simulink model "Integration4"  (R2025a)
settings: Solver=ode113  StartTime=0.0  StopTime=7200  FixedStep=1e-04  MaxStep=72  RelTol=1e-3
libraries: simulink x3302
(part 1 of 141)
settings Model: Creator=kbiswas  LastModifiedBy=kaust
settings RTWCC: GPUComputeCapability=3.5

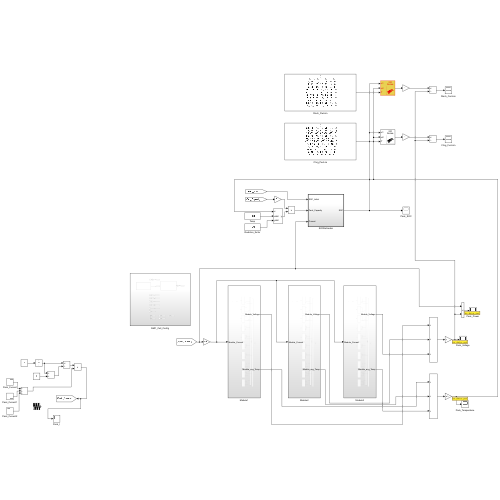
[thumbnail: Simulink's stored preview of the top-level diagram]
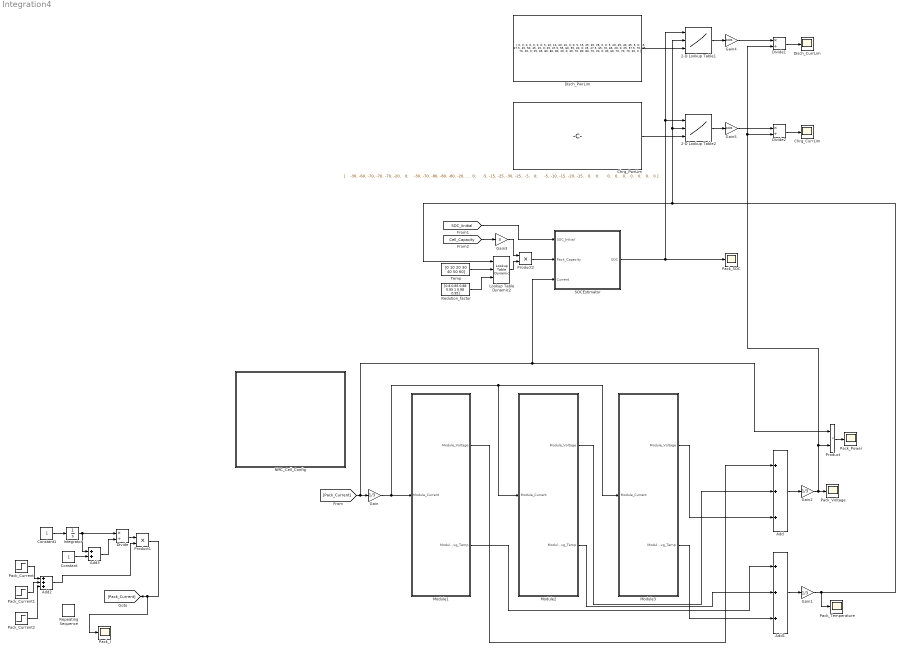
== system Integration4 ==
  2-D Lookup Table1 : Lookup_n-D  LookupTableObject=''  BreakpointsForDimension1=[0 0.1 0.2 0.3 0.4 0.5 0.6 0.7 0.8 0.9 1]  BreakpointsForDimension2=[0 10 20 30 40 50 60]  BreakpointsForDimension1FirstPoint=10  BreakpointsForDimension2FirstPoint=10  BreakpointsForDimension1Spacing=12  BreakpointsForDimension2Spacing=12  IndexSearchMethod=Evenly spaced points  TableSource=Input port  Table=|  InterpMethod=Akima spline  DiagnosticForOutOfRangeInput=Error  InternalRulePriority=Speed  RndMeth=Simplest
      | [
      |     2.954364, 3.109857, 3.273534, 3.3066, 3.34,    3.3734,  3.20473;
      |     3.122427, 3.286765, 3.459753, 3.4947, 3.53,    3.5653,  3.387035;
      |     3.175499, 3.342631, 3.518559, 3.5541, 3.59,    3.6259,  3.444605;
      |     3.210881, 3.379875, 3.557763, 3.5937, 3.63,    3.6663,  3.482985;
      |     3.237417, 3.407808, 3.587166, 3.6234, 3.66,    3.6966,  3.511777;
      |     3.272799, 3.445052, 3.62637,  3.663,  3.7,     3.737,   3.55015;
      |     3.317026, 3.491066, 3.675375, 3.7125, 3.75,    3.7875,  3.598125;
      |     3.387789, 3.566094, 3.753783, 3.7917, 3.83,    3.8683,  3.674885;
      |     3.467398, 3.649892, 3.841992, 3.8808, 3.92,    3.9592,  3.76124;
      |     3.564697, 3.752313, 3.949803, 3.9897, 4.03,    4.0703,  3.866785;
      |     3.653151, 3.845422, 4.047813, 4.0887, 4.13,    4.1713,  3.962735
      | ]
      settings: InputPortMap=u0,u1,p221
  2-D Lookup Table2 : Lookup_n-D  LookupTableObject=''  BreakpointsForDimension1=[0 0.1 0.2 0.3 0.4 0.5 0.6 0.7 0.8 0.9 1]  BreakpointsForDimension2=[0 10 20 30 40 50 60]  BreakpointsForDimension1FirstPoint=10  BreakpointsForDimension2FirstPoint=10  BreakpointsForDimension1Spacing=12  BreakpointsForDimension2Spacing=12  IndexSearchMethod=Evenly spaced points  TableSource=Input port  Table=|  InterpMethod=Akima spline  DiagnosticForOutOfRangeInput=Error  InternalRulePriority=Speed  RndMeth=Simplest
      | [
      |     2.954364, 3.109857, 3.273534, 3.3066, 3.34,    3.3734,  3.20473;
      |     3.122427, 3.286765, 3.459753, 3.4947, 3.53,    3.5653,  3.387035;
      |     3.175499, 3.342631, 3.518559, 3.5541, 3.59,    3.6259,  3.444605;
      |     3.210881, 3.379875, 3.557763, 3.5937, 3.63,    3.6663,  3.482985;
      |     3.237417, 3.407808, 3.587166, 3.6234, 3.66,    3.6966,  3.511777;
      |     3.272799, 3.445052, 3.62637,  3.663,  3.7,     3.737,   3.55015;
      |     3.317026, 3.491066, 3.675375, 3.7125, 3.75,    3.7875,  3.598125;
      |     3.387789, 3.566094, 3.753783, 3.7917, 3.83,    3.8683,  3.674885;
      |     3.467398, 3.649892, 3.841992, 3.8808, 3.92,    3.9592,  3.76124;
      |     3.564697, 3.752313, 3.949803, 3.9897, 4.03,    4.0703,  3.866785;
      |     3.653151, 3.845422, 4.047813, 4.0887, 4.13,    4.1713,  3.962735
      | ]
      settings: InputPortMap=u0,u1,p221
  Add : Sum  Inputs=+++
  Add1 : Sum  Inputs=+++
  Add2 : Sum  Inputs=+++
  Add3 : Sum
  Chrg_CurrLim : Scope
      settings: ActiveDisplayYMinimum=-0.029859398179627156  ActiveDisplayYMaximum=1.1144288220199585  DataLoggingVariableName=ScopeData8
  Chrg_PwrLim : Constant  Value=|
      | [
      |    -30, -60, -70, -70, -70, -20,   0;
      |    -30, -70, -80, -80, -80, -20,   0;
      |    -25, -65, -80, -80, -80, -20,   0;
      |    -25, -55, -70, -75, -70, -20,   0;
      |    -25, -47.5, -65, -70, -65, -20,  0;
      |    -25, -37.5, -55, -60, -55, -20,  0;
      |    -15, -27.5, -45, -50, -45, -15,  0;
      |     -5, -20, -35, -40, -35,  -5,   0;
      |     -5, -15, -25, -30, -25,  -5,   0;
      |     -5, -10, -15, -20, -15,   0,   0;
      |      0,   0,   0,   0,   0,   0,   0
      | ]
  Constant : Constant
  Constant1 : Constant
  Disch_CurrLim : Scope
      settings: ActiveDisplayYMinimum=-0.029859398179627156  ActiveDisplayYMaximum=1.1144288220199585  DataLoggingVariableName=ScopeData7
  Disch_PwrLim : Constant  Value=|
      | [
      |      0,   0,   0,   0,   0,   0,   0;
      |      5,  10,  10,  20,  10,   0,   0;
      |      5,  15,  25,  30,  25,   5,   0;
      |      5,  20,  35,  40,  35,   5,   0;
      |     15, 27.5, 45,  50,  45,  15,   0;
      |     25, 37.5, 55,  60,  55,  20,   0;
      |     25, 47.5, 65,  70,  65,  20,   0;
      |     25, 57.5, 70,  75,  70,  20,   0;
      |     25, 65,   80,  80,  80,  20,   0;
      |     30, 70,   80,  80,  70,  20,   0;
      |     30, 60,   70,  70,  70,  20,   0
      | ]
  Divide : Product  Inputs=*/
  Divide1 : Product  Inputs=*/
  Divide2 : Product  Inputs=*/
  Gain : Gain  Gain=1/3
  Gain1 : Gain  Gain=1/3
  Gain2 : Gain  Gain=1/3
  Gain3 : Gain  Gain=3
  Gain4 : Gain  Gain=1000
  Gain5 : Gain  Gain=1000
  Integrator : Integrator
  Lookup Table Dynamic2 : simulink/Lookup Tables/Lookup Table Dynamic  LookUpMeth=Interpolation-Use End Values  OutDataType=fixdt('double')  OutScaling=[]  OutputDataTypeScalingMode=Specify via dialog  OutDataTypeStr=fixdt('double')  DoSatur=off
  Module1 : Subsystem
  Module2 : Subsystem
  Module3 : Subsystem
  NMC_Cell_Config : Subsystem
  Pack_Current : Step  After=70  SampleTime=0
  Pack_Current1 : Step  Time=3601  After=-70  SampleTime=0
  Pack_Current2 : Step  Time=3610  After=-70  SampleTime=0
  Pack_I : Scope
      settings: ActiveDisplayYMinimum=-87.4866348128896  ActiveDisplayYMaximum=87.47692203701736  DataLoggingVariableName=ScopeData5
  Pack_Power : Scope
      settings: ActiveDisplayYMinimum=-86878.920066941544  ActiveDisplayYMaximum=76635.6657175614  DataLoggingVariableName=ScopeData4
  Pack_SOC : Scope
      settings: ActiveDisplayYMinimum=-0.029859398179627156  ActiveDisplayYMaximum=1.1144288220199585  DataLoggingVariableName=ScopeData6
  Pack_Temperature : Scope
      settings: ActiveDisplayYMinimum=24.036198918147498  ActiveDisplayYMaximum=33.674209736672459  DataLoggingVariableName=ScopeData2
  Pack_Voltage : Scope
      settings: ActiveDisplayYMinimum=715.78941909752871  ActiveDisplayYMaximum=961.19940125009657
  Product : Product
  Product1 : Product
  Product2 : Product
  Redution_factor : Constant  Value=[0.8 0.85 0.88 0.95 1 0.98 0.95]
  Repeating Sequence : simulink/Sources/Repeating Sequence  rep_seq_t=[0 200 400 600 800]  rep_seq_y=[0 70 0 -70 0]
  SOCEstimator : Subsystem  TreatAsAtomicUnit=on
  Temp : Constant  Value=[0 10 20 30 40 50 60]
  wires:
  [Pack_Current] -> Product/1, SOCEstimator/3(Current), Gain/1
  Gain/1 -> Module2/1(Module_Current), Module3/1(Module_Current), Module1/1(Module_Current)
  Module1/1(Module_Voltage) -> Add/1
  Module2/1(Module_Voltage) -> Add/2
  Module3/1(Module_Voltage) -> Add/3
  Module1/2(Module_avg_Temp) -> Add1/1
  Module2/2(Module_avg_Temp) -> Add1/2
  Module3/2(Module_avg_Temp) -> Add1/3
  Add1/1 -> Gain1/1
  Add/1 -> Gain2/1
  Gain2/1 -> Divide2/2, Divide1/2, Product/2, Pack_Voltage/1
  Pack_Current/1 -> Add2/1
  Pack_Current1/1 -> Add2/2
  Product/1 -> Pack_Power/1
  Product1/1 -> Pack_I/1, [Pack_Current]
  Add2/1 -> Product1/2
  Integrator/1 -> Divide/1, Add3/1
  Constant/1 -> Add3/2
  Add3/1 -> Divide/2
  Constant1/1 -> Integrator/1
  Divide/1 -> Product1/1
  Pack_Current2/1 -> Add2/3
  [SOC_Iinitial] -> SOCEstimator/1(SOC_Initial)
  Lookup Table Dynamic2/1 -> Product2/2
  [Cell_Capacity] -> Gain3/1
  Temp/1 -> Lookup Table Dynamic2/2
  Gain1/1 -> 2-D Lookup Table1/2, 2-D Lookup Table2/2, Lookup Table Dynamic2/1, Pack_Temperature/1
  Redution_factor/1 -> Lookup Table Dynamic2/3
  Product2/1 -> SOCEstimator/2(Pack_Capacity)
  Gain3/1 -> Product2/1
  SOCEstimator/1(SOC) -> 2-D Lookup Table2/1, 2-D Lookup Table1/1, Pack_SOC/1
  Disch_PwrLim/1 -> 2-D Lookup Table1/3
  Chrg_PwrLim/1 -> 2-D Lookup Table2/3
  2-D Lookup Table1/1 -> Gain4/1
  2-D Lookup Table2/1 -> Gain5/1
  Gain4/1 -> Divide1/1
  Gain5/1 -> Divide2/1
  Divide1/1 -> Disch_CurrLim/1
  Divide2/1 -> Chrg_CurrLim/1

== system Integration4/Module1 ==
  Module_Current : Inport
  Add : Sum  Inputs=++++++++++
  Add1 : Sum  Inputs=++++++++++
  Constant : Constant  Value=10
  Divide : Product  Inputs=*/
  Scope : Scope
      settings: ActiveDisplayYMinimum=675.19968  ActiveDisplayYMaximum=920.25224
  Scope1 : Scope
      settings: ActiveDisplayYMinimum=23.92172  ActiveDisplayYMaximum=34.70451  DataLoggingVariableName=ScopeData3
  SubModule_1 : Subsystem
  SubModule_10 : Subsystem
  SubModule_2 : Subsystem
  SubModule_3 : Subsystem
  SubModule_4 : Subsystem
  SubModule_5 : Subsystem
  SubModule_6 : Subsystem
  SubModule_7 : Subsystem
  SubModule_8 : Subsystem
  SubModule_9 : Subsystem
  Module_Voltage : Outport
  Module_avg_Temp : Outport  Port=2
  wires:
  SubModule_4/2(SubModule_avg_temp) -> Add1/4
  Add/1 -> Module_Voltage/1, Scope/1
  [Module_Current] -> SubModule_5/1(Module_Current)
  [Module_Current] -> SubModule_9/1(Module_Current)
  [Module_Current] -> SubModule_2/1(Module_Current)
  [Module_Current] -> SubModule_3/1(Module_Current)
  [Module_Current] -> SubModule_7/1(Module_Current)
  Module_Current/1 -> [Module_Current]
  SubModule_1/1(SubModule_Voltage) -> Add/1
  [Module_Current] -> SubModule_1/1(Module_Current)
  [Module_Current] -> SubModule_4/1(Module_Current)
  SubModule_6/2(SubModule_avg_temp) -> Add1/6
  Divide/1 -> Module_avg_Temp/1, Scope1/1
  SubModule_5/1(SubModule_Voltage) -> Add/5
  [Module_Current] -> SubModule_8/1(Module_Current)
  SubModule_8/2(SubModule_avg_temp) -> Add1/8
  SubModule_5/2(SubModule_avg_temp) -> Add1/5
  SubModule_8/1(SubModule_Voltage) -> Add/8
  [Module_Current] -> SubModule_10/1(Module_Current)
  Constant/1 -> Divide/2
  SubModule_10/1(SubModule_Voltage) -> Add/10
  SubModule_10/2(SubModule_avg_temp) -> Add1/10
  SubModule_7/1(SubModule_Voltage) -> Add/7
  SubModule_9/2(SubModule_avg_temp) -> Add1/9
  SubModule_3/1(SubModule_Voltage) -> Add/3
  SubModule_4/1(SubModule_Voltage) -> Add/4
  SubModule_2/2(SubModule_avg_temp) -> Add1/2
  SubModule_3/2(SubModule_avg_temp) -> Add1/3
  SubModule_7/2(SubModule_avg_temp) -> Add1/7
  Add1/1 -> Divide/1
  SubModule_9/1(SubModule_Voltage) -> Add/9
  SubModule_6/1(SubModule_Voltage) -> Add/6
  SubModule_2/1(SubModule_Voltage) -> Add/2
  SubModule_1/2(SubModule_avg_temp) -> Add1/1
  [Module_Current] -> SubModule_6/1(Module_Current)

== system Integration4/Module2 ==
  Module_Current : Inport
  Add : Sum  Inputs=++++++++++
  Add1 : Sum  Inputs=++++++++++
  Constant : Constant  Value=10
  Divide : Product  Inputs=*/
  Scope : Scope
      settings: ActiveDisplayYMinimum=675.19968  ActiveDisplayYMaximum=920.25224
  Scope1 : Scope
      settings: ActiveDisplayYMinimum=23.92172  ActiveDisplayYMaximum=34.70451  DataLoggingVariableName=ScopeData3
  SubModule_1 : Subsystem
  SubModule_10 : Subsystem
  SubModule_2 : Subsystem
  SubModule_3 : Subsystem
  SubModule_4 : Subsystem
  SubModule_5 : Subsystem
  SubModule_6 : Subsystem
  SubModule_7 : Subsystem
  SubModule_8 : Subsystem
  SubModule_9 : Subsystem
  Module_Voltage : Outport
  Module_avg_Temp : Outport  Port=2
  wires:
  SubModule_4/2(SubModule_avg_temp) -> Add1/4
  Add/1 -> Module_Voltage/1, Scope/1
  [Module_Current] -> SubModule_5/1(Module_Current)
  [Module_Current] -> SubModule_9/1(Module_Current)
  [Module_Current] -> SubModule_2/1(Module_Current)
  [Module_Current] -> SubModule_3/1(Module_Current)
  [Module_Current] -> SubModule_7/1(Module_Current)
  Module_Current/1 -> [Module_Current]
  SubModule_1/1(SubModule_Voltage) -> Add/1
  [Module_Current] -> SubModule_1/1(Module_Current)
  [Module_Current] -> SubModule_4/1(Module_Current)
  SubModule_6/2(SubModule_avg_temp) -> Add1/6
  Divide/1 -> Module_avg_Temp/1, Scope1/1
  SubModule_5/1(SubModule_Voltage) -> Add/5
  [Module_Current] -> SubModule_8/1(Module_Current)
  SubModule_8/2(SubModule_avg_temp) -> Add1/8
  SubModule_5/2(SubModule_avg_temp) -> Add1/5
  SubModule_8/1(SubModule_Voltage) -> Add/8
  [Module_Current] -> SubModule_10/1(Module_Current)
  Constant/1 -> Divide/2
  SubModule_10/1(SubModule_Voltage) -> Add/10
  SubModule_10/2(SubModule_avg_temp) -> Add1/10
  SubModule_7/1(SubModule_Voltage) -> Add/7
  SubModule_9/2(SubModule_avg_temp) -> Add1/9
  SubModule_3/1(SubModule_Voltage) -> Add/3
  SubModule_4/1(SubModule_Voltage) -> Add/4
  SubModule_2/2(SubModule_avg_temp) -> Add1/2
  SubModule_3/2(SubModule_avg_temp) -> Add1/3
  SubModule_7/2(SubModule_avg_temp) -> Add1/7
  Add1/1 -> Divide/1
  SubModule_9/1(SubModule_Voltage) -> Add/9
  SubModule_6/1(SubModule_Voltage) -> Add/6
  SubModule_2/1(SubModule_Voltage) -> Add/2
  SubModule_1/2(SubModule_avg_temp) -> Add1/1
  [Module_Current] -> SubModule_6/1(Module_Current)

== system Integration4/Module3 ==
  Module_Current : Inport
  Add : Sum  Inputs=++++++++++
  Add1 : Sum  Inputs=++++++++++
  Constant : Constant  Value=10
  Divide : Product  Inputs=*/
  Scope : Scope
      settings: ActiveDisplayYMinimum=618.46252  ActiveDisplayYMaximum=926.55637
  Scope1 : Scope
      settings: ActiveDisplayYMinimum=23.92172  ActiveDisplayYMaximum=34.70451  DataLoggingVariableName=ScopeData3
  SubModule_1 : Subsystem
  SubModule_10 : Subsystem
  SubModule_2 : Subsystem
  SubModule_3 : Subsystem
  SubModule_4 : Subsystem
  SubModule_5 : Subsystem
  SubModule_6 : Subsystem
  SubModule_7 : Subsystem
  SubModule_8 : Subsystem
  SubModule_9 : Subsystem
  Module_Voltage : Outport
  Module_avg_Temp : Outport  Port=2
  wires:
  [Module_Current] -> SubModule_6/1(Module_Current)
  SubModule_1/2(SubModule_avg_temp) -> Add1/1
  SubModule_2/1(SubModule_Voltage) -> Add/2
  SubModule_6/1(SubModule_Voltage) -> Add/6
  SubModule_9/1(SubModule_Voltage) -> Add/9
  Add1/1 -> Divide/1
  SubModule_7/2(SubModule_avg_temp) -> Add1/7
  SubModule_3/2(SubModule_avg_temp) -> Add1/3
  SubModule_2/2(SubModule_avg_temp) -> Add1/2
  SubModule_4/1(SubModule_Voltage) -> Add/4
  SubModule_3/1(SubModule_Voltage) -> Add/3
  SubModule_9/2(SubModule_avg_temp) -> Add1/9
  SubModule_7/1(SubModule_Voltage) -> Add/7
  SubModule_10/2(SubModule_avg_temp) -> Add1/10
  SubModule_10/1(SubModule_Voltage) -> Add/10
  Constant/1 -> Divide/2
  [Module_Current] -> SubModule_10/1(Module_Current)
  SubModule_8/1(SubModule_Voltage) -> Add/8
  SubModule_5/2(SubModule_avg_temp) -> Add1/5
  SubModule_8/2(SubModule_avg_temp) -> Add1/8
  [Module_Current] -> SubModule_8/1(Module_Current)
  SubModule_5/1(SubModule_Voltage) -> Add/5
  Divide/1 -> Scope1/1, Module_avg_Temp/1
  SubModule_6/2(SubModule_avg_temp) -> Add1/6
  [Module_Current] -> SubModule_4/1(Module_Current)
  [Module_Current] -> SubModule_1/1(Module_Current)
  SubModule_1/1(SubModule_Voltage) -> Add/1
  Module_Current/1 -> [Module_Current]
  [Module_Current] -> SubModule_7/1(Module_Current)
  [Module_Current] -> SubModule_3/1(Module_Current)
  [Module_Current] -> SubModule_2/1(Module_Current)
  [Module_Current] -> SubModule_9/1(Module_Current)
  [Module_Current] -> SubModule_5/1(Module_Current)
  Add/1 -> Scope/1, Module_Voltage/1
  SubModule_4/2(SubModule_avg_temp) -> Add1/4

== system Integration4/NMC_Cell_Config ==
  A : Constant  Value=0.013
  C1_User1 : Constant  Value=[800 850 900 950 1000 1050 1000 950 900 850 800]
  C2_User : Constant  Value=[15 16 17 18 19 20 19 18 17 16 15]
  Cell_Capacity_Ah_rated : Constant  Value=26.5
  Gain1 : Gain  Gain=1e-03
  Gain2 : Gain
  Gain3 : Gain  Gain=1e-03
  Gain4 : Gain  Gain=1e+03
  Gain5 : Gain  Gain=0.01
  Gain6 : Gain  Gain=1e-04
  Goto11 : Goto  TagVisibility=global
  M*Cp : Constant  Value=369
  OCV_NMC : Constant  Value=|
      | [
      |     2.954364, 3.109857, 3.273534, 3.3066, 3.34,    3.3734,  3.20473;
      |     3.122427, 3.286765, 3.459753, 3.4947, 3.53,    3.5653,  3.387035;
      |     3.175499, 3.342631, 3.518559, 3.5541, 3.59,    3.6259,  3.444605;
      |     3.210881, 3.379875, 3.557763, 3.5937, 3.63,    3.6663,  3.482985;
      |     3.237417, 3.407808, 3.587166, 3.6234, 3.66,    3.6966,  3.511777;
      |     3.272799, 3.445052, 3.62637,  3.663,  3.7,     3.737,   3.55015;
      |     3.317026, 3.491066, 3.675375, 3.7125, 3.75,    3.7875,  3.598125;
      |     3.387789, 3.566094, 3.753783, 3.7917, 3.83,    3.8683,  3.674885;
      |     3.467398, 3.649892, 3.841992, 3.8808, 3.92,    3.9592,  3.76124;
      |     3.564697, 3.752313, 3.949803, 3.9897, 4.03,    4.0703,  3.866785;
      |     3.653151, 3.845422, 4.047813, 4.0887, 4.13,    4.1713,  3.962735
      | ]
  R1_User : Constant  Value=[1.5 1.2 0.9 0.7 0.6 0.5 0.5 0.5 0.6 0.7 0.8]
  R2_User1 : Constant  Value=[2.5 2 1.6 1.3 1.1 1 1.1 1.2 1.3 1.4 1.5]
  Ri_NMC : Constant  Value=|
      | [67.2155, 61.105, 55.55, 55, 52.25, 49.6375, 54.60125;
      |     48.884, 44.44, 40.4, 40, 38, 36.1, 39.71;
      |     44.60665, 40.5515, 36.865, 36.5, 34.675, 32.94125, 36.23538;
      |     41.5514, 37.774, 34.34, 34, 32.83, 30.685, 33.7535;
      |     40.3293, 36.663, 33.33, 33, 31.35, 29.7825, 32.76075;
      |     39.71825, 36.1075, 32.825, 32.5, 31.25, 29.33125, 32.26438;
      |     40.08488, 36.4408, 33.128, 32.8, 31.16, 29.602, 32.5622;
      |     40.94035, 37.2185, 33.835, 33.5, 31.825, 30.23375, 33.15738;
      |     42.7735, 38.1925, 35.03, 34.7, 32.375, 31.5875, 34.74263;
      |     51.3282, 46.602, 42.42, 42, 39.9, 37.905, 41.6955;
      |     73.326, 66.66, 60.6, 60, 57, 54.15, 59.565]
  SOC_Initial_% : Constant  Value=100
  SOC_User : Constant  Value=[0 10 20 30 40 50 60 70 80 90 100]
  Temp_Initial_degC : Constant  Value=25
  Temp_ambient : Constant  Value=25
  h : Constant  Value=20
  tag scope: C1_User=global, C2_User=global, Cell_Capacity=global, Cp=global, OCV=global, R1_User=global, R2_User=global, Ri_User=global, SOC_Iinitial=global, SOC_User=global, Temp_Iinitial=global, Temp_ambient=global, h=global
  wires:
  OCV_NMC/1 -> [OCV]
  SOC_User/1 -> Gain5/1
  R1_User/1 -> Gain1/1
  Gain1/1 -> [R1_User]
  C1_User1/1 -> Gain2/1
  Gain2/1 -> [C1_User]
  R2_User1/1 -> Gain3/1
  Gain3/1 -> [R2_User]
  Gain4/1 -> [C2_User]
  C2_User/1 -> Gain4/1
  Cell_Capacity_Ah_rated/1 -> [Cell_Capacity]
  SOC_Initial_%/1 -> [SOC_Iinitial]
  Gain5/1 -> [SOC_User]
  Temp_Initial_degC/1 -> [Temp_ambient], [Temp_Iinitial]
  h/1 -> [h]
  A/1 -> Goto11/1
  M*Cp/1 -> [Cp]
  Gain6/1 -> [Ri_User]
  Ri_NMC/1 -> Gain6/1

== system Integration4/SOCEstimator ==
  SOC_Initial : Inport
  Pack_Capacity : Inport  Port=2
  Current : Inport  Port=3
  SOCEstimator : Subsystem
  SOC : Outport
  wires:
  SOCEstimator/1(SOC) -> SOC/1
  SOC_Initial/1 -> SOCEstimator/1(SOC_Initial)
  Current/1 -> SOCEstimator/2(Current)
  Pack_Capacity/1 -> SOCEstimator/3(CellCapacity)

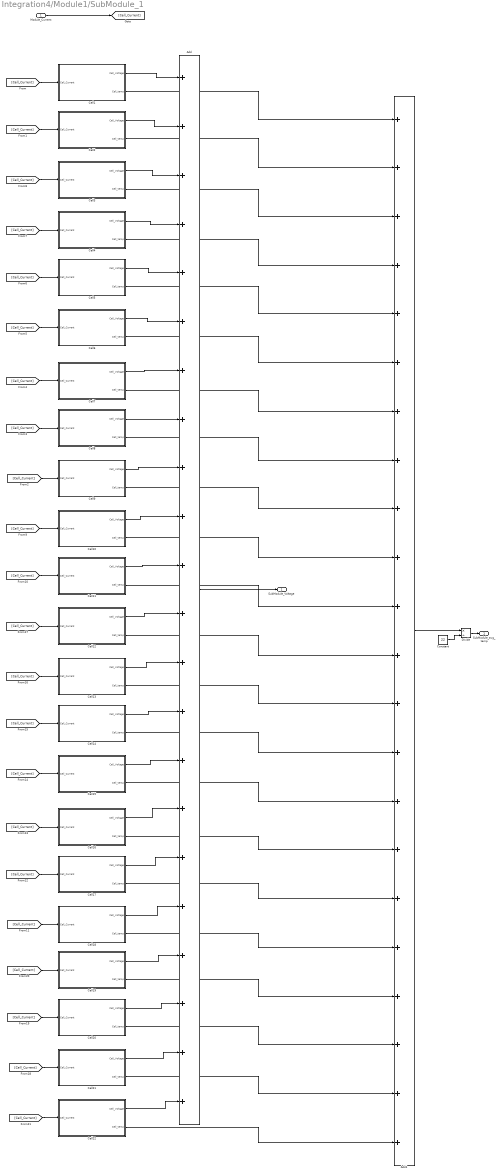
== system Integration4/Module1/SubModule_1 ==
  Module_Current : Inport
  Add : Sum  Inputs=++++++++++++++++++++++
  Add1 : Sum  Inputs=++++++++++++++++++++++
  Cell1 : Subsystem
  Cell10 : Subsystem
  Cell11 : Subsystem
  Cell12 : Subsystem
  Cell13 : Subsystem
  Cell14 : Subsystem
  Cell15 : Subsystem
  Cell16 : Subsystem
  Cell17 : Subsystem
  Cell18 : Subsystem
  Cell19 : Subsystem
  Cell2 : Subsystem
  Cell20 : Subsystem
  Cell21 : Subsystem
  Cell22 : Subsystem
  Cell3 : Subsystem
  Cell4 : Subsystem
  Cell5 : Subsystem
  Cell6 : Subsystem
  Cell7 : Subsystem
  Cell8 : Subsystem
  Cell9 : Subsystem
  Constant : Constant  Value=22
  Divide : Product  Inputs=*/
  SubModule_Voltage : Outport
  SubModule_avg_temp : Outport  Port=2
  wires:
  Cell9/2(Cell_temp) -> Add1/9
  [Cell_Current] -> Cell8/1(Cell_Current)
  Cell13/1(Cell_Voltage) -> Add/13
  Cell4/1(Cell_Voltage) -> Add/4
  Module_Current/1 -> [Cell_Current]
  Cell15/1(Cell_Voltage) -> Add/15
  [Cell_Current] -> Cell7/1(Cell_Current)
  [Cell_Current] -> Cell10/1(Cell_Current)
  Cell21/2(Cell_temp) -> Add1/21
  Cell5/1(Cell_Voltage) -> Add/5
  [Cell_Current] -> Cell1/1(Cell_Current)
  Cell2/1(Cell_Voltage) -> Add/2
  Cell19/1(Cell_Voltage) -> Add/19
  [Cell_Current] -> Cell5/1(Cell_Current)
  [Cell_Current] -> Cell11/1(Cell_Current)
  Cell6/1(Cell_Voltage) -> Add/6
  Cell11/1(Cell_Voltage) -> Add/11
  [Cell_Current] -> Cell18/1(Cell_Current)
  Cell7/2(Cell_temp) -> Add1/7
  [Cell_Current] -> Cell21/1(Cell_Current)
  [Cell_Current] -> Cell12/1(Cell_Current)
  [Cell_Current] -> Cell4/1(Cell_Current)
  Cell18/1(Cell_Voltage) -> Add/18
  Cell20/1(Cell_Voltage) -> Add/20
  Cell11/2(Cell_temp) -> Add1/11
  [Cell_Current] -> Cell2/1(Cell_Current)
  Cell16/2(Cell_temp) -> Add1/16
  [Cell_Current] -> Cell15/1(Cell_Current)
  [Cell_Current] -> Cell6/1(Cell_Current)
  [Cell_Current] -> Cell13/1(Cell_Current)
  Cell2/2(Cell_temp) -> Add1/2
  Cell22/2(Cell_temp) -> Add1/22
  Cell9/1(Cell_Voltage) -> Add/9
  Cell7/1(Cell_Voltage) -> Add/7
  [Cell_Current] -> Cell9/1(Cell_Current)
  Cell14/2(Cell_temp) -> Add1/14
  Cell17/1(Cell_Voltage) -> Add/17
  Cell10/2(Cell_temp) -> Add1/10
  [Cell_Current] -> Cell16/1(Cell_Current)
  Cell8/1(Cell_Voltage) -> Add/8
  Cell21/1(Cell_Voltage) -> Add/21
  Cell12/2(Cell_temp) -> Add1/12
  Cell22/1(Cell_Voltage) -> Add/22
  [Cell_Current] -> Cell20/1(Cell_Current)
  [Cell_Current] -> Cell17/1(Cell_Current)
  Cell10/1(Cell_Voltage) -> Add/10
  Cell18/2(Cell_temp) -> Add1/18
  Cell14/1(Cell_Voltage) -> Add/14
  Cell16/1(Cell_Voltage) -> Add/16
  [Cell_Current] -> Cell3/1(Cell_Current)
  Cell12/1(Cell_Voltage) -> Add/12
  Cell20/2(Cell_temp) -> Add1/20
  Cell1/1(Cell_Voltage) -> Add/1
  [Cell_Current] -> Cell19/1(Cell_Current)
  Cell3/1(Cell_Voltage) -> Add/3
  [Cell_Current] -> Cell22/1(Cell_Current)
  [Cell_Current] -> Cell14/1(Cell_Current)
  Cell19/2(Cell_temp) -> Add1/19
  Cell6/2(Cell_temp) -> Add1/6
  Cell17/2(Cell_temp) -> Add1/17
  Cell15/2(Cell_temp) -> Add1/15
  Cell8/2(Cell_temp) -> Add1/8
  Cell3/2(Cell_temp) -> Add1/3
  Cell13/2(Cell_temp) -> Add1/13
  Add/1 -> SubModule_Voltage/1
  Cell4/2(Cell_temp) -> Add1/4
  Cell5/2(Cell_temp) -> Add1/5
  Cell1/2(Cell_temp) -> Add1/1
  Add1/1 -> Divide/1
  Constant/1 -> Divide/2
  Divide/1 -> SubModule_avg_temp/1

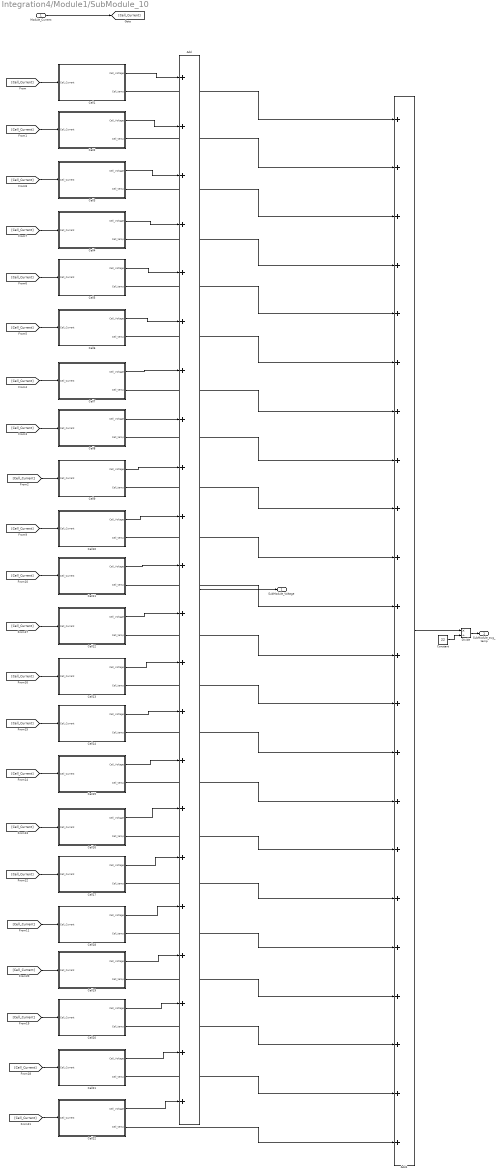
== system Integration4/Module1/SubModule_10 ==
  Module_Current : Inport
  Add : Sum  Inputs=++++++++++++++++++++++
  Add1 : Sum  Inputs=++++++++++++++++++++++
  Cell1 : Subsystem
  Cell10 : Subsystem
  Cell11 : Subsystem
  Cell12 : Subsystem
  Cell13 : Subsystem
  Cell14 : Subsystem
  Cell15 : Subsystem
  Cell16 : Subsystem
  Cell17 : Subsystem
  Cell18 : Subsystem
  Cell19 : Subsystem
  Cell2 : Subsystem
  Cell20 : Subsystem
  Cell21 : Subsystem
  Cell22 : Subsystem
  Cell3 : Subsystem
  Cell4 : Subsystem
  Cell5 : Subsystem
  Cell6 : Subsystem
  Cell7 : Subsystem
  Cell8 : Subsystem
  Cell9 : Subsystem
  Constant : Constant  Value=22
  Divide : Product  Inputs=*/
  SubModule_Voltage : Outport
  SubModule_avg_temp : Outport  Port=2
  wires:
  Cell9/2(Cell_temp) -> Add1/9
  [Cell_Current] -> Cell8/1(Cell_Current)
  Cell13/1(Cell_Voltage) -> Add/13
  Cell4/1(Cell_Voltage) -> Add/4
  Module_Current/1 -> [Cell_Current]
  Cell15/1(Cell_Voltage) -> Add/15
  [Cell_Current] -> Cell7/1(Cell_Current)
  [Cell_Current] -> Cell10/1(Cell_Current)
  Cell21/2(Cell_temp) -> Add1/21
  Cell5/1(Cell_Voltage) -> Add/5
  [Cell_Current] -> Cell1/1(Cell_Current)
  Cell2/1(Cell_Voltage) -> Add/2
  Cell19/1(Cell_Voltage) -> Add/19
  [Cell_Current] -> Cell5/1(Cell_Current)
  [Cell_Current] -> Cell11/1(Cell_Current)
  Cell6/1(Cell_Voltage) -> Add/6
  Cell11/1(Cell_Voltage) -> Add/11
  [Cell_Current] -> Cell18/1(Cell_Current)
  Cell7/2(Cell_temp) -> Add1/7
  [Cell_Current] -> Cell21/1(Cell_Current)
  [Cell_Current] -> Cell12/1(Cell_Current)
  [Cell_Current] -> Cell4/1(Cell_Current)
  Cell18/1(Cell_Voltage) -> Add/18
  Cell20/1(Cell_Voltage) -> Add/20
  Cell11/2(Cell_temp) -> Add1/11
  [Cell_Current] -> Cell2/1(Cell_Current)
  Cell16/2(Cell_temp) -> Add1/16
  [Cell_Current] -> Cell15/1(Cell_Current)
  [Cell_Current] -> Cell6/1(Cell_Current)
  [Cell_Current] -> Cell13/1(Cell_Current)
  Cell2/2(Cell_temp) -> Add1/2
  Cell22/2(Cell_temp) -> Add1/22
  Cell9/1(Cell_Voltage) -> Add/9
  Cell7/1(Cell_Voltage) -> Add/7
  [Cell_Current] -> Cell9/1(Cell_Current)
  Cell14/2(Cell_temp) -> Add1/14
  Cell17/1(Cell_Voltage) -> Add/17
  Cell10/2(Cell_temp) -> Add1/10
  [Cell_Current] -> Cell16/1(Cell_Current)
  Cell8/1(Cell_Voltage) -> Add/8
  Cell21/1(Cell_Voltage) -> Add/21
  Cell12/2(Cell_temp) -> Add1/12
  Cell22/1(Cell_Voltage) -> Add/22
  [Cell_Current] -> Cell20/1(Cell_Current)
  [Cell_Current] -> Cell17/1(Cell_Current)
  Cell10/1(Cell_Voltage) -> Add/10
  Cell18/2(Cell_temp) -> Add1/18
  Cell14/1(Cell_Voltage) -> Add/14
  Cell16/1(Cell_Voltage) -> Add/16
  [Cell_Current] -> Cell3/1(Cell_Current)
  Cell12/1(Cell_Voltage) -> Add/12
  Cell20/2(Cell_temp) -> Add1/20
  Cell1/1(Cell_Voltage) -> Add/1
  [Cell_Current] -> Cell19/1(Cell_Current)
  Cell3/1(Cell_Voltage) -> Add/3
  [Cell_Current] -> Cell22/1(Cell_Current)
  [Cell_Current] -> Cell14/1(Cell_Current)
  Cell19/2(Cell_temp) -> Add1/19
  Cell6/2(Cell_temp) -> Add1/6
  Cell17/2(Cell_temp) -> Add1/17
  Cell15/2(Cell_temp) -> Add1/15
  Cell8/2(Cell_temp) -> Add1/8
  Cell3/2(Cell_temp) -> Add1/3
  Cell13/2(Cell_temp) -> Add1/13
  Add/1 -> SubModule_Voltage/1
  Cell4/2(Cell_temp) -> Add1/4
  Cell5/2(Cell_temp) -> Add1/5
  Cell1/2(Cell_temp) -> Add1/1
  Add1/1 -> Divide/1
  Constant/1 -> Divide/2
  Divide/1 -> SubModule_avg_temp/1

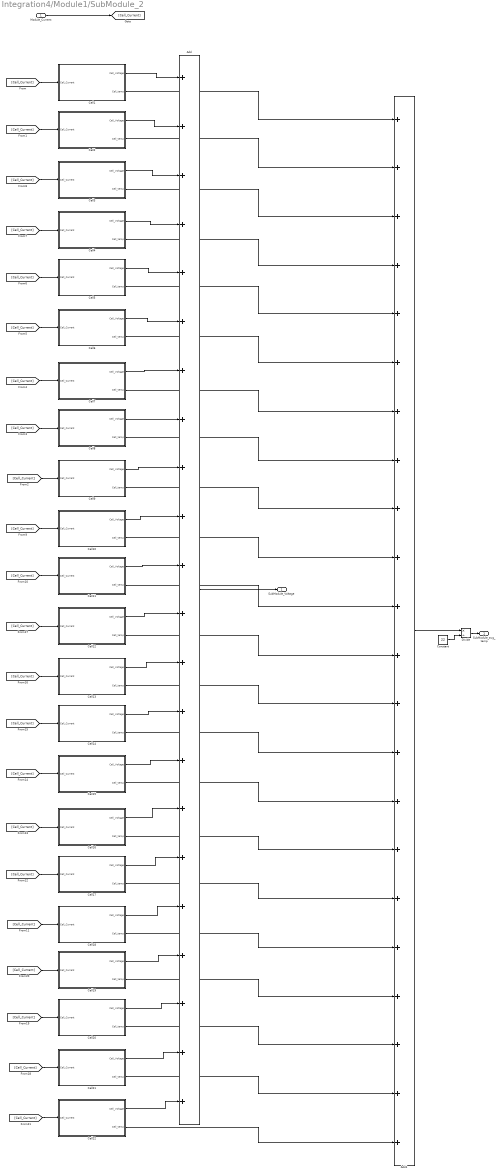
== system Integration4/Module1/SubModule_2 ==
  Module_Current : Inport
  Add : Sum  Inputs=++++++++++++++++++++++
  Add1 : Sum  Inputs=++++++++++++++++++++++
  Cell1 : Subsystem
  Cell10 : Subsystem
  Cell11 : Subsystem
  Cell12 : Subsystem
  Cell13 : Subsystem
  Cell14 : Subsystem
  Cell15 : Subsystem
  Cell16 : Subsystem
  Cell17 : Subsystem
  Cell18 : Subsystem
  Cell19 : Subsystem
  Cell2 : Subsystem
  Cell20 : Subsystem
  Cell21 : Subsystem
  Cell22 : Subsystem
  Cell3 : Subsystem
  Cell4 : Subsystem
  Cell5 : Subsystem
  Cell6 : Subsystem
  Cell7 : Subsystem
  Cell8 : Subsystem
  Cell9 : Subsystem
  Constant : Constant  Value=22
  Divide : Product  Inputs=*/
  SubModule_Voltage : Outport
  SubModule_avg_temp : Outport  Port=2
  wires:
  Divide/1 -> SubModule_avg_temp/1
  Constant/1 -> Divide/2
  Add1/1 -> Divide/1
  Cell1/2(Cell_temp) -> Add1/1
  Cell5/2(Cell_temp) -> Add1/5
  Cell4/2(Cell_temp) -> Add1/4
  Add/1 -> SubModule_Voltage/1
  Cell13/2(Cell_temp) -> Add1/13
  Cell3/2(Cell_temp) -> Add1/3
  Cell8/2(Cell_temp) -> Add1/8
  Cell15/2(Cell_temp) -> Add1/15
  Cell17/2(Cell_temp) -> Add1/17
  Cell6/2(Cell_temp) -> Add1/6
  Cell19/2(Cell_temp) -> Add1/19
  [Cell_Current] -> Cell14/1(Cell_Current)
  [Cell_Current] -> Cell22/1(Cell_Current)
  Cell3/1(Cell_Voltage) -> Add/3
  [Cell_Current] -> Cell19/1(Cell_Current)
  Cell1/1(Cell_Voltage) -> Add/1
  Cell20/2(Cell_temp) -> Add1/20
  Cell12/1(Cell_Voltage) -> Add/12
  [Cell_Current] -> Cell3/1(Cell_Current)
  Cell16/1(Cell_Voltage) -> Add/16
  Cell14/1(Cell_Voltage) -> Add/14
  Cell18/2(Cell_temp) -> Add1/18
  Cell10/1(Cell_Voltage) -> Add/10
  [Cell_Current] -> Cell17/1(Cell_Current)
  [Cell_Current] -> Cell20/1(Cell_Current)
  Cell22/1(Cell_Voltage) -> Add/22
  Cell12/2(Cell_temp) -> Add1/12
  Cell21/1(Cell_Voltage) -> Add/21
  Cell8/1(Cell_Voltage) -> Add/8
  [Cell_Current] -> Cell16/1(Cell_Current)
  Cell10/2(Cell_temp) -> Add1/10
  Cell17/1(Cell_Voltage) -> Add/17
  Cell14/2(Cell_temp) -> Add1/14
  [Cell_Current] -> Cell9/1(Cell_Current)
  Cell7/1(Cell_Voltage) -> Add/7
  Cell9/1(Cell_Voltage) -> Add/9
  Cell22/2(Cell_temp) -> Add1/22
  Cell2/2(Cell_temp) -> Add1/2
  [Cell_Current] -> Cell13/1(Cell_Current)
  [Cell_Current] -> Cell6/1(Cell_Current)
  [Cell_Current] -> Cell15/1(Cell_Current)
  Cell16/2(Cell_temp) -> Add1/16
  [Cell_Current] -> Cell2/1(Cell_Current)
  Cell11/2(Cell_temp) -> Add1/11
  Cell20/1(Cell_Voltage) -> Add/20
  Cell18/1(Cell_Voltage) -> Add/18
  [Cell_Current] -> Cell4/1(Cell_Current)
  [Cell_Current] -> Cell12/1(Cell_Current)
  [Cell_Current] -> Cell21/1(Cell_Current)
  Cell7/2(Cell_temp) -> Add1/7
  [Cell_Current] -> Cell18/1(Cell_Current)
  Cell11/1(Cell_Voltage) -> Add/11
  Cell6/1(Cell_Voltage) -> Add/6
  [Cell_Current] -> Cell11/1(Cell_Current)
  [Cell_Current] -> Cell5/1(Cell_Current)
  Cell19/1(Cell_Voltage) -> Add/19
  Cell2/1(Cell_Voltage) -> Add/2
  [Cell_Current] -> Cell1/1(Cell_Current)
  Cell5/1(Cell_Voltage) -> Add/5
  Cell21/2(Cell_temp) -> Add1/21
  [Cell_Current] -> Cell10/1(Cell_Current)
  [Cell_Current] -> Cell7/1(Cell_Current)
  Cell15/1(Cell_Voltage) -> Add/15
  Module_Current/1 -> [Cell_Current]
  Cell4/1(Cell_Voltage) -> Add/4
  Cell13/1(Cell_Voltage) -> Add/13
  [Cell_Current] -> Cell8/1(Cell_Current)
  Cell9/2(Cell_temp) -> Add1/9

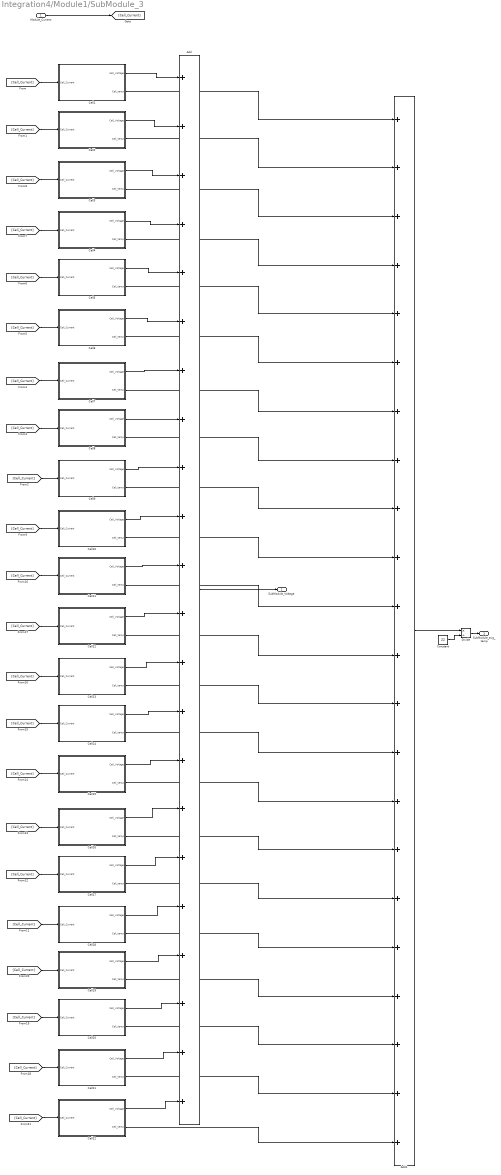
== system Integration4/Module1/SubModule_3 ==
  Module_Current : Inport
  Add : Sum  Inputs=++++++++++++++++++++++
  Add1 : Sum  Inputs=++++++++++++++++++++++
  Cell1 : Subsystem
  Cell10 : Subsystem
  Cell11 : Subsystem
  Cell12 : Subsystem
  Cell13 : Subsystem
  Cell14 : Subsystem
  Cell15 : Subsystem
  Cell16 : Subsystem
  Cell17 : Subsystem
  Cell18 : Subsystem
  Cell19 : Subsystem
  Cell2 : Subsystem
  Cell20 : Subsystem
  Cell21 : Subsystem
  Cell22 : Subsystem
  Cell3 : Subsystem
  Cell4 : Subsystem
  Cell5 : Subsystem
  Cell6 : Subsystem
  Cell7 : Subsystem
  Cell8 : Subsystem
  Cell9 : Subsystem
  Constant : Constant  Value=22
  Divide : Product  Inputs=*/
  SubModule_Voltage : Outport
  SubModule_avg_temp : Outport  Port=2
  wires:
  Cell9/2(Cell_temp) -> Add1/9
  [Cell_Current] -> Cell8/1(Cell_Current)
  Cell13/1(Cell_Voltage) -> Add/13
  Cell4/1(Cell_Voltage) -> Add/4
  Module_Current/1 -> [Cell_Current]
  Cell15/1(Cell_Voltage) -> Add/15
  [Cell_Current] -> Cell7/1(Cell_Current)
  [Cell_Current] -> Cell10/1(Cell_Current)
  Cell21/2(Cell_temp) -> Add1/21
  Cell5/1(Cell_Voltage) -> Add/5
  [Cell_Current] -> Cell1/1(Cell_Current)
  Cell2/1(Cell_Voltage) -> Add/2
  Cell19/1(Cell_Voltage) -> Add/19
  [Cell_Current] -> Cell5/1(Cell_Current)
  [Cell_Current] -> Cell11/1(Cell_Current)
  Cell6/1(Cell_Voltage) -> Add/6
  Cell11/1(Cell_Voltage) -> Add/11
  [Cell_Current] -> Cell18/1(Cell_Current)
  Cell7/2(Cell_temp) -> Add1/7
  [Cell_Current] -> Cell21/1(Cell_Current)
  [Cell_Current] -> Cell12/1(Cell_Current)
  [Cell_Current] -> Cell4/1(Cell_Current)
  Cell18/1(Cell_Voltage) -> Add/18
  Cell20/1(Cell_Voltage) -> Add/20
  Cell11/2(Cell_temp) -> Add1/11
  [Cell_Current] -> Cell2/1(Cell_Current)
  Cell16/2(Cell_temp) -> Add1/16
  [Cell_Current] -> Cell15/1(Cell_Current)
  [Cell_Current] -> Cell6/1(Cell_Current)
  [Cell_Current] -> Cell13/1(Cell_Current)
  Cell2/2(Cell_temp) -> Add1/2
  Cell22/2(Cell_temp) -> Add1/22
  Cell9/1(Cell_Voltage) -> Add/9
  Cell7/1(Cell_Voltage) -> Add/7
  [Cell_Current] -> Cell9/1(Cell_Current)
  Cell14/2(Cell_temp) -> Add1/14
  Cell17/1(Cell_Voltage) -> Add/17
  Cell10/2(Cell_temp) -> Add1/10
  [Cell_Current] -> Cell16/1(Cell_Current)
  Cell8/1(Cell_Voltage) -> Add/8
  Cell21/1(Cell_Voltage) -> Add/21
  Cell12/2(Cell_temp) -> Add1/12
  Cell22/1(Cell_Voltage) -> Add/22
  [Cell_Current] -> Cell20/1(Cell_Current)
  [Cell_Current] -> Cell17/1(Cell_Current)
  Cell10/1(Cell_Voltage) -> Add/10
  Cell18/2(Cell_temp) -> Add1/18
  Cell14/1(Cell_Voltage) -> Add/14
  Cell16/1(Cell_Voltage) -> Add/16
  [Cell_Current] -> Cell3/1(Cell_Current)
  Cell12/1(Cell_Voltage) -> Add/12
  Cell20/2(Cell_temp) -> Add1/20
  Cell1/1(Cell_Voltage) -> Add/1
  [Cell_Current] -> Cell19/1(Cell_Current)
  Cell3/1(Cell_Voltage) -> Add/3
  [Cell_Current] -> Cell22/1(Cell_Current)
  [Cell_Current] -> Cell14/1(Cell_Current)
  Cell19/2(Cell_temp) -> Add1/19
  Cell6/2(Cell_temp) -> Add1/6
  Cell17/2(Cell_temp) -> Add1/17
  Cell15/2(Cell_temp) -> Add1/15
  Cell8/2(Cell_temp) -> Add1/8
  Cell3/2(Cell_temp) -> Add1/3
  Cell13/2(Cell_temp) -> Add1/13
  Add/1 -> SubModule_Voltage/1
  Cell4/2(Cell_temp) -> Add1/4
  Cell5/2(Cell_temp) -> Add1/5
  Cell1/2(Cell_temp) -> Add1/1
  Add1/1 -> Divide/1
  Constant/1 -> Divide/2
  Divide/1 -> SubModule_avg_temp/1

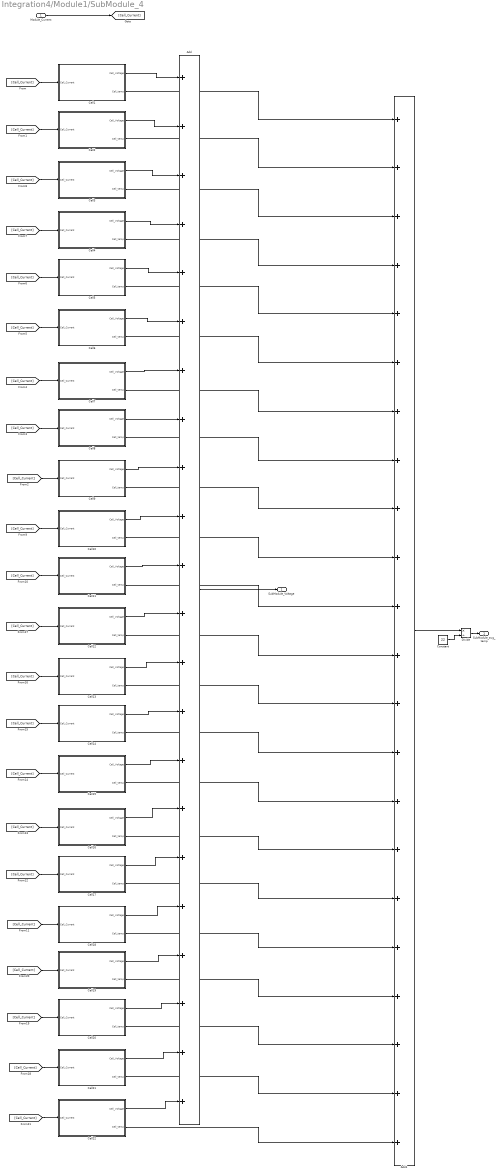
== system Integration4/Module1/SubModule_4 ==
  Module_Current : Inport
  Add : Sum  Inputs=++++++++++++++++++++++
  Add1 : Sum  Inputs=++++++++++++++++++++++
  Cell1 : Subsystem
  Cell10 : Subsystem
  Cell11 : Subsystem
  Cell12 : Subsystem
  Cell13 : Subsystem
  Cell14 : Subsystem
  Cell15 : Subsystem
  Cell16 : Subsystem
  Cell17 : Subsystem
  Cell18 : Subsystem
  Cell19 : Subsystem
  Cell2 : Subsystem
  Cell20 : Subsystem
  Cell21 : Subsystem
  Cell22 : Subsystem
  Cell3 : Subsystem
  Cell4 : Subsystem
  Cell5 : Subsystem
  Cell6 : Subsystem
  Cell7 : Subsystem
  Cell8 : Subsystem
  Cell9 : Subsystem
  Constant : Constant  Value=22
  Divide : Product  Inputs=*/
  SubModule_Voltage : Outport
  SubModule_avg_temp : Outport  Port=2
  wires:
  Divide/1 -> SubModule_avg_temp/1
  Constant/1 -> Divide/2
  Add1/1 -> Divide/1
  Cell1/2(Cell_temp) -> Add1/1
  Cell5/2(Cell_temp) -> Add1/5
  Cell4/2(Cell_temp) -> Add1/4
  Add/1 -> SubModule_Voltage/1
  Cell13/2(Cell_temp) -> Add1/13
  Cell3/2(Cell_temp) -> Add1/3
  Cell8/2(Cell_temp) -> Add1/8
  Cell15/2(Cell_temp) -> Add1/15
  Cell17/2(Cell_temp) -> Add1/17
  Cell6/2(Cell_temp) -> Add1/6
  Cell19/2(Cell_temp) -> Add1/19
  [Cell_Current] -> Cell14/1(Cell_Current)
  [Cell_Current] -> Cell22/1(Cell_Current)
  Cell3/1(Cell_Voltage) -> Add/3
  [Cell_Current] -> Cell19/1(Cell_Current)
  Cell1/1(Cell_Voltage) -> Add/1
  Cell20/2(Cell_temp) -> Add1/20
  Cell12/1(Cell_Voltage) -> Add/12
  [Cell_Current] -> Cell3/1(Cell_Current)
  Cell16/1(Cell_Voltage) -> Add/16
  Cell14/1(Cell_Voltage) -> Add/14
  Cell18/2(Cell_temp) -> Add1/18
  Cell10/1(Cell_Voltage) -> Add/10
  [Cell_Current] -> Cell17/1(Cell_Current)
  [Cell_Current] -> Cell20/1(Cell_Current)
  Cell22/1(Cell_Voltage) -> Add/22
  Cell12/2(Cell_temp) -> Add1/12
  Cell21/1(Cell_Voltage) -> Add/21
  Cell8/1(Cell_Voltage) -> Add/8
  [Cell_Current] -> Cell16/1(Cell_Current)
  Cell10/2(Cell_temp) -> Add1/10
  Cell17/1(Cell_Voltage) -> Add/17
  Cell14/2(Cell_temp) -> Add1/14
  [Cell_Current] -> Cell9/1(Cell_Current)
  Cell7/1(Cell_Voltage) -> Add/7
  Cell9/1(Cell_Voltage) -> Add/9
  Cell22/2(Cell_temp) -> Add1/22
  Cell2/2(Cell_temp) -> Add1/2
  [Cell_Current] -> Cell13/1(Cell_Current)
  [Cell_Current] -> Cell6/1(Cell_Current)
  [Cell_Current] -> Cell15/1(Cell_Current)
  Cell16/2(Cell_temp) -> Add1/16
  [Cell_Current] -> Cell2/1(Cell_Current)
  Cell11/2(Cell_temp) -> Add1/11
  Cell20/1(Cell_Voltage) -> Add/20
  Cell18/1(Cell_Voltage) -> Add/18
  [Cell_Current] -> Cell4/1(Cell_Current)
  [Cell_Current] -> Cell12/1(Cell_Current)
  [Cell_Current] -> Cell21/1(Cell_Current)
  Cell7/2(Cell_temp) -> Add1/7
  [Cell_Current] -> Cell18/1(Cell_Current)
  Cell11/1(Cell_Voltage) -> Add/11
  Cell6/1(Cell_Voltage) -> Add/6
  [Cell_Current] -> Cell11/1(Cell_Current)
  [Cell_Current] -> Cell5/1(Cell_Current)
  Cell19/1(Cell_Voltage) -> Add/19
  Cell2/1(Cell_Voltage) -> Add/2
  [Cell_Current] -> Cell1/1(Cell_Current)
  Cell5/1(Cell_Voltage) -> Add/5
  Cell21/2(Cell_temp) -> Add1/21
  [Cell_Current] -> Cell10/1(Cell_Current)
  [Cell_Current] -> Cell7/1(Cell_Current)
  Cell15/1(Cell_Voltage) -> Add/15
  Module_Current/1 -> [Cell_Current]
  Cell4/1(Cell_Voltage) -> Add/4
  Cell13/1(Cell_Voltage) -> Add/13
  [Cell_Current] -> Cell8/1(Cell_Current)
  Cell9/2(Cell_temp) -> Add1/9

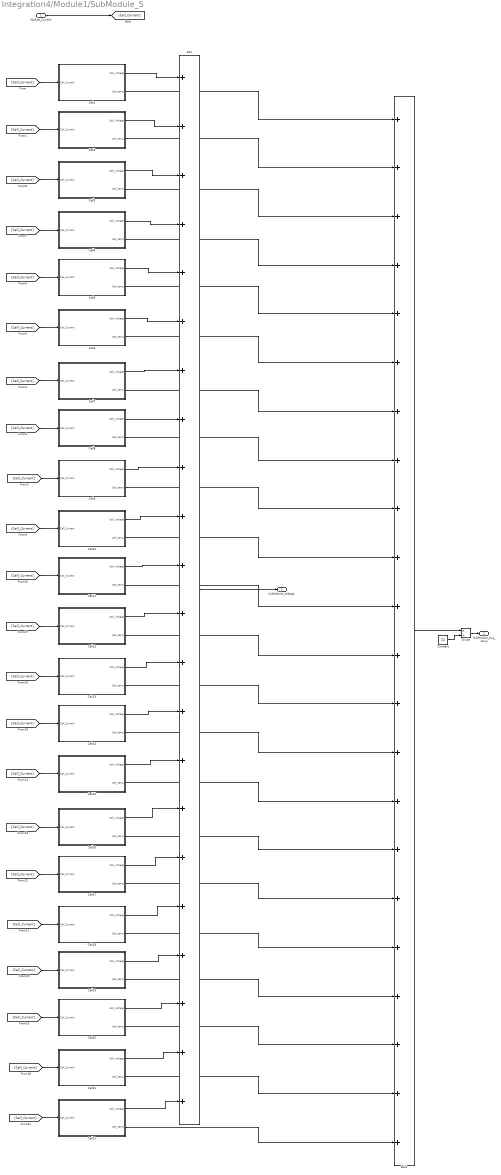
== system Integration4/Module1/SubModule_5 ==
  Module_Current : Inport
  Add : Sum  Inputs=++++++++++++++++++++++
  Add1 : Sum  Inputs=++++++++++++++++++++++
  Cell1 : Subsystem
  Cell10 : Subsystem
  Cell11 : Subsystem
  Cell12 : Subsystem
  Cell13 : Subsystem
  Cell14 : Subsystem
  Cell15 : Subsystem
  Cell16 : Subsystem
  Cell17 : Subsystem
  Cell18 : Subsystem
  Cell19 : Subsystem
  Cell2 : Subsystem
  Cell20 : Subsystem
  Cell21 : Subsystem
  Cell22 : Subsystem
  Cell3 : Subsystem
  Cell4 : Subsystem
  Cell5 : Subsystem
  Cell6 : Subsystem
  Cell7 : Subsystem
  Cell8 : Subsystem
  Cell9 : Subsystem
  Constant : Constant  Value=22
  Divide : Product  Inputs=*/
  SubModule_Voltage : Outport
  SubModule_avg_temp : Outport  Port=2
  wires:
  Cell9/2(Cell_temp) -> Add1/9
  [Cell_Current] -> Cell8/1(Cell_Current)
  Cell13/1(Cell_Voltage) -> Add/13
  Cell4/1(Cell_Voltage) -> Add/4
  Module_Current/1 -> [Cell_Current]
  Cell15/1(Cell_Voltage) -> Add/15
  [Cell_Current] -> Cell7/1(Cell_Current)
  [Cell_Current] -> Cell10/1(Cell_Current)
  Cell21/2(Cell_temp) -> Add1/21
  Cell5/1(Cell_Voltage) -> Add/5
  [Cell_Current] -> Cell1/1(Cell_Current)
  Cell2/1(Cell_Voltage) -> Add/2
  Cell19/1(Cell_Voltage) -> Add/19
  [Cell_Current] -> Cell5/1(Cell_Current)
  [Cell_Current] -> Cell11/1(Cell_Current)
  Cell6/1(Cell_Voltage) -> Add/6
  Cell11/1(Cell_Voltage) -> Add/11
  [Cell_Current] -> Cell18/1(Cell_Current)
  Cell7/2(Cell_temp) -> Add1/7
  [Cell_Current] -> Cell21/1(Cell_Current)
  [Cell_Current] -> Cell12/1(Cell_Current)
  [Cell_Current] -> Cell4/1(Cell_Current)
  Cell18/1(Cell_Voltage) -> Add/18
  Cell20/1(Cell_Voltage) -> Add/20
  Cell11/2(Cell_temp) -> Add1/11
  [Cell_Current] -> Cell2/1(Cell_Current)
  Cell16/2(Cell_temp) -> Add1/16
  [Cell_Current] -> Cell15/1(Cell_Current)
  [Cell_Current] -> Cell6/1(Cell_Current)
  [Cell_Current] -> Cell13/1(Cell_Current)
  Cell2/2(Cell_temp) -> Add1/2
  Cell22/2(Cell_temp) -> Add1/22
  Cell9/1(Cell_Voltage) -> Add/9
  Cell7/1(Cell_Voltage) -> Add/7
  [Cell_Current] -> Cell9/1(Cell_Current)
  Cell14/2(Cell_temp) -> Add1/14
  Cell17/1(Cell_Voltage) -> Add/17
  Cell10/2(Cell_temp) -> Add1/10
  [Cell_Current] -> Cell16/1(Cell_Current)
  Cell8/1(Cell_Voltage) -> Add/8
  Cell21/1(Cell_Voltage) -> Add/21
  Cell12/2(Cell_temp) -> Add1/12
  Cell22/1(Cell_Voltage) -> Add/22
  [Cell_Current] -> Cell20/1(Cell_Current)
  [Cell_Current] -> Cell17/1(Cell_Current)
  Cell10/1(Cell_Voltage) -> Add/10
  Cell18/2(Cell_temp) -> Add1/18
  Cell14/1(Cell_Voltage) -> Add/14
  Cell16/1(Cell_Voltage) -> Add/16
  [Cell_Current] -> Cell3/1(Cell_Current)
  Cell12/1(Cell_Voltage) -> Add/12
  Cell20/2(Cell_temp) -> Add1/20
  Cell1/1(Cell_Voltage) -> Add/1
  [Cell_Current] -> Cell19/1(Cell_Current)
  Cell3/1(Cell_Voltage) -> Add/3
  [Cell_Current] -> Cell22/1(Cell_Current)
  [Cell_Current] -> Cell14/1(Cell_Current)
  Cell19/2(Cell_temp) -> Add1/19
  Cell6/2(Cell_temp) -> Add1/6
  Cell17/2(Cell_temp) -> Add1/17
  Cell15/2(Cell_temp) -> Add1/15
  Cell8/2(Cell_temp) -> Add1/8
  Cell3/2(Cell_temp) -> Add1/3
  Cell13/2(Cell_temp) -> Add1/13
  Add/1 -> SubModule_Voltage/1
  Cell4/2(Cell_temp) -> Add1/4
  Cell5/2(Cell_temp) -> Add1/5
  Cell1/2(Cell_temp) -> Add1/1
  Add1/1 -> Divide/1
  Constant/1 -> Divide/2
  Divide/1 -> SubModule_avg_temp/1

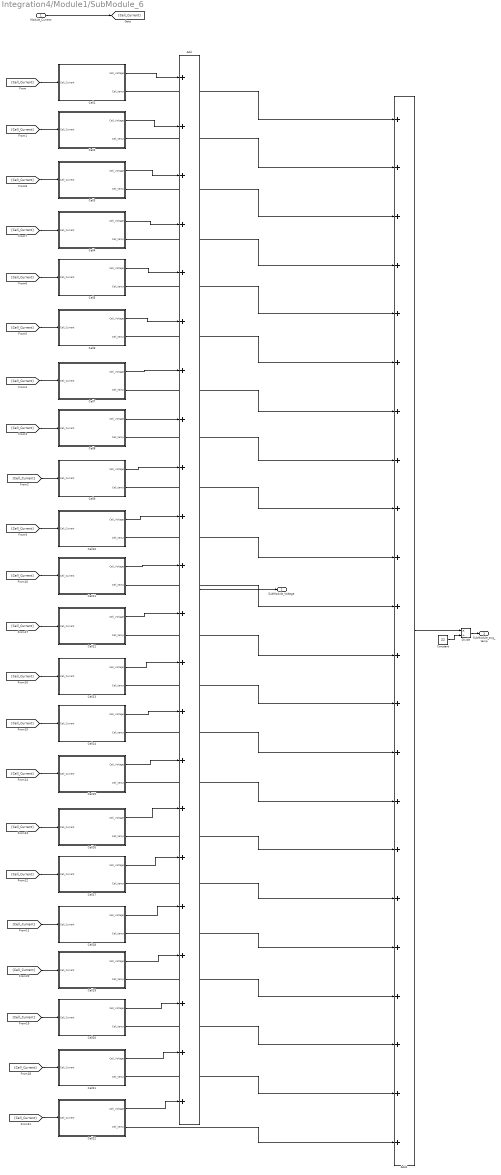
== system Integration4/Module1/SubModule_6 ==
  Module_Current : Inport
  Add : Sum  Inputs=++++++++++++++++++++++
  Add1 : Sum  Inputs=++++++++++++++++++++++
  Cell1 : Subsystem
  Cell10 : Subsystem
  Cell11 : Subsystem
  Cell12 : Subsystem
  Cell13 : Subsystem
  Cell14 : Subsystem
  Cell15 : Subsystem
  Cell16 : Subsystem
  Cell17 : Subsystem
  Cell18 : Subsystem
  Cell19 : Subsystem
  Cell2 : Subsystem
  Cell20 : Subsystem
  Cell21 : Subsystem
  Cell22 : Subsystem
  Cell3 : Subsystem
  Cell4 : Subsystem
  Cell5 : Subsystem
  Cell6 : Subsystem
  Cell7 : Subsystem
  Cell8 : Subsystem
  Cell9 : Subsystem
  Constant : Constant  Value=22
  Divide : Product  Inputs=*/
  SubModule_Voltage : Outport
  SubModule_avg_temp : Outport  Port=2
  wires:
  Divide/1 -> SubModule_avg_temp/1
  Constant/1 -> Divide/2
  Add1/1 -> Divide/1
  Cell1/2(Cell_temp) -> Add1/1
  Cell5/2(Cell_temp) -> Add1/5
  Cell4/2(Cell_temp) -> Add1/4
  Add/1 -> SubModule_Voltage/1
  Cell13/2(Cell_temp) -> Add1/13
  Cell3/2(Cell_temp) -> Add1/3
  Cell8/2(Cell_temp) -> Add1/8
  Cell15/2(Cell_temp) -> Add1/15
  Cell17/2(Cell_temp) -> Add1/17
  Cell6/2(Cell_temp) -> Add1/6
  Cell19/2(Cell_temp) -> Add1/19
  [Cell_Current] -> Cell14/1(Cell_Current)
  [Cell_Current] -> Cell22/1(Cell_Current)
  Cell3/1(Cell_Voltage) -> Add/3
  [Cell_Current] -> Cell19/1(Cell_Current)
  Cell1/1(Cell_Voltage) -> Add/1
  Cell20/2(Cell_temp) -> Add1/20
  Cell12/1(Cell_Voltage) -> Add/12
  [Cell_Current] -> Cell3/1(Cell_Current)
  Cell16/1(Cell_Voltage) -> Add/16
  Cell14/1(Cell_Voltage) -> Add/14
  Cell18/2(Cell_temp) -> Add1/18
  Cell10/1(Cell_Voltage) -> Add/10
  [Cell_Current] -> Cell17/1(Cell_Current)
  [Cell_Current] -> Cell20/1(Cell_Current)
  Cell22/1(Cell_Voltage) -> Add/22
  Cell12/2(Cell_temp) -> Add1/12
  Cell21/1(Cell_Voltage) -> Add/21
  Cell8/1(Cell_Voltage) -> Add/8
  [Cell_Current] -> Cell16/1(Cell_Current)
  Cell10/2(Cell_temp) -> Add1/10
  Cell17/1(Cell_Voltage) -> Add/17
  Cell14/2(Cell_temp) -> Add1/14
  [Cell_Current] -> Cell9/1(Cell_Current)
  Cell7/1(Cell_Voltage) -> Add/7
  Cell9/1(Cell_Voltage) -> Add/9
  Cell22/2(Cell_temp) -> Add1/22
  Cell2/2(Cell_temp) -> Add1/2
  [Cell_Current] -> Cell13/1(Cell_Current)
  [Cell_Current] -> Cell6/1(Cell_Current)
  [Cell_Current] -> Cell15/1(Cell_Current)
  Cell16/2(Cell_temp) -> Add1/16
  [Cell_Current] -> Cell2/1(Cell_Current)
  Cell11/2(Cell_temp) -> Add1/11
  Cell20/1(Cell_Voltage) -> Add/20
  Cell18/1(Cell_Voltage) -> Add/18
  [Cell_Current] -> Cell4/1(Cell_Current)
  [Cell_Current] -> Cell12/1(Cell_Current)
  [Cell_Current] -> Cell21/1(Cell_Current)
  Cell7/2(Cell_temp) -> Add1/7
  [Cell_Current] -> Cell18/1(Cell_Current)
  Cell11/1(Cell_Voltage) -> Add/11
  Cell6/1(Cell_Voltage) -> Add/6
  [Cell_Current] -> Cell11/1(Cell_Current)
  [Cell_Current] -> Cell5/1(Cell_Current)
  Cell19/1(Cell_Voltage) -> Add/19
  Cell2/1(Cell_Voltage) -> Add/2
  [Cell_Current] -> Cell1/1(Cell_Current)
  Cell5/1(Cell_Voltage) -> Add/5
  Cell21/2(Cell_temp) -> Add1/21
  [Cell_Current] -> Cell10/1(Cell_Current)
  [Cell_Current] -> Cell7/1(Cell_Current)
  Cell15/1(Cell_Voltage) -> Add/15
  Module_Current/1 -> [Cell_Current]
  Cell4/1(Cell_Voltage) -> Add/4
  Cell13/1(Cell_Voltage) -> Add/13
  [Cell_Current] -> Cell8/1(Cell_Current)
  Cell9/2(Cell_temp) -> Add1/9

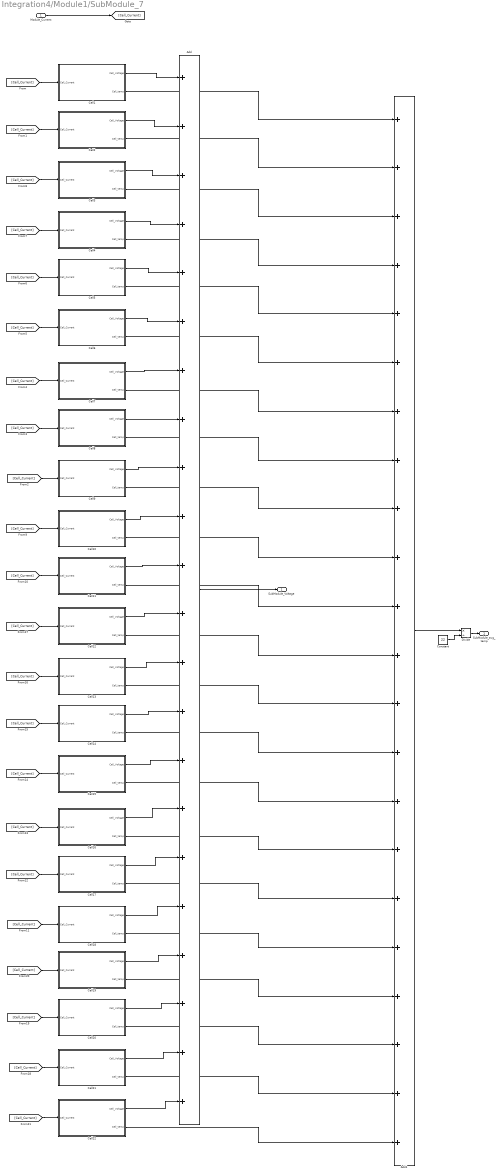
== system Integration4/Module1/SubModule_7 ==
  Module_Current : Inport
  Add : Sum  Inputs=++++++++++++++++++++++
  Add1 : Sum  Inputs=++++++++++++++++++++++
  Cell1 : Subsystem
  Cell10 : Subsystem
  Cell11 : Subsystem
  Cell12 : Subsystem
  Cell13 : Subsystem
  Cell14 : Subsystem
  Cell15 : Subsystem
  Cell16 : Subsystem
  Cell17 : Subsystem
  Cell18 : Subsystem
  Cell19 : Subsystem
  Cell2 : Subsystem
  Cell20 : Subsystem
  Cell21 : Subsystem
  Cell22 : Subsystem
  Cell3 : Subsystem
  Cell4 : Subsystem
  Cell5 : Subsystem
  Cell6 : Subsystem
  Cell7 : Subsystem
  Cell8 : Subsystem
  Cell9 : Subsystem
  Constant : Constant  Value=22
  Divide : Product  Inputs=*/
  SubModule_Voltage : Outport
  SubModule_avg_temp : Outport  Port=2
  wires:
  Divide/1 -> SubModule_avg_temp/1
  Constant/1 -> Divide/2
  Add1/1 -> Divide/1
  Cell1/2(Cell_temp) -> Add1/1
  Cell5/2(Cell_temp) -> Add1/5
  Cell4/2(Cell_temp) -> Add1/4
  Add/1 -> SubModule_Voltage/1
  Cell13/2(Cell_temp) -> Add1/13
  Cell3/2(Cell_temp) -> Add1/3
  Cell8/2(Cell_temp) -> Add1/8
  Cell15/2(Cell_temp) -> Add1/15
  Cell17/2(Cell_temp) -> Add1/17
  Cell6/2(Cell_temp) -> Add1/6
  Cell19/2(Cell_temp) -> Add1/19
  [Cell_Current] -> Cell14/1(Cell_Current)
  [Cell_Current] -> Cell22/1(Cell_Current)
  Cell3/1(Cell_Voltage) -> Add/3
  [Cell_Current] -> Cell19/1(Cell_Current)
  Cell1/1(Cell_Voltage) -> Add/1
  Cell20/2(Cell_temp) -> Add1/20
  Cell12/1(Cell_Voltage) -> Add/12
  [Cell_Current] -> Cell3/1(Cell_Current)
  Cell16/1(Cell_Voltage) -> Add/16
  Cell14/1(Cell_Voltage) -> Add/14
  Cell18/2(Cell_temp) -> Add1/18
  Cell10/1(Cell_Voltage) -> Add/10
  [Cell_Current] -> Cell17/1(Cell_Current)
  [Cell_Current] -> Cell20/1(Cell_Current)
  Cell22/1(Cell_Voltage) -> Add/22
  Cell12/2(Cell_temp) -> Add1/12
  Cell21/1(Cell_Voltage) -> Add/21
  Cell8/1(Cell_Voltage) -> Add/8
  [Cell_Current] -> Cell16/1(Cell_Current)
  Cell10/2(Cell_temp) -> Add1/10
  Cell17/1(Cell_Voltage) -> Add/17
  Cell14/2(Cell_temp) -> Add1/14
  [Cell_Current] -> Cell9/1(Cell_Current)
  Cell7/1(Cell_Voltage) -> Add/7
  Cell9/1(Cell_Voltage) -> Add/9
  Cell22/2(Cell_temp) -> Add1/22
  Cell2/2(Cell_temp) -> Add1/2
  [Cell_Current] -> Cell13/1(Cell_Current)
  [Cell_Current] -> Cell6/1(Cell_Current)
  [Cell_Current] -> Cell15/1(Cell_Current)
  Cell16/2(Cell_temp) -> Add1/16
  [Cell_Current] -> Cell2/1(Cell_Current)
  Cell11/2(Cell_temp) -> Add1/11
  Cell20/1(Cell_Voltage) -> Add/20
  Cell18/1(Cell_Voltage) -> Add/18
  [Cell_Current] -> Cell4/1(Cell_Current)
  [Cell_Current] -> Cell12/1(Cell_Current)
  [Cell_Current] -> Cell21/1(Cell_Current)
  Cell7/2(Cell_temp) -> Add1/7
  [Cell_Current] -> Cell18/1(Cell_Current)
  Cell11/1(Cell_Voltage) -> Add/11
  Cell6/1(Cell_Voltage) -> Add/6
  [Cell_Current] -> Cell11/1(Cell_Current)
  [Cell_Current] -> Cell5/1(Cell_Current)
  Cell19/1(Cell_Voltage) -> Add/19
  Cell2/1(Cell_Voltage) -> Add/2
  [Cell_Current] -> Cell1/1(Cell_Current)
  Cell5/1(Cell_Voltage) -> Add/5
  Cell21/2(Cell_temp) -> Add1/21
  [Cell_Current] -> Cell10/1(Cell_Current)
  [Cell_Current] -> Cell7/1(Cell_Current)
  Cell15/1(Cell_Voltage) -> Add/15
  Module_Current/1 -> [Cell_Current]
  Cell4/1(Cell_Voltage) -> Add/4
  Cell13/1(Cell_Voltage) -> Add/13
  [Cell_Current] -> Cell8/1(Cell_Current)
  Cell9/2(Cell_temp) -> Add1/9

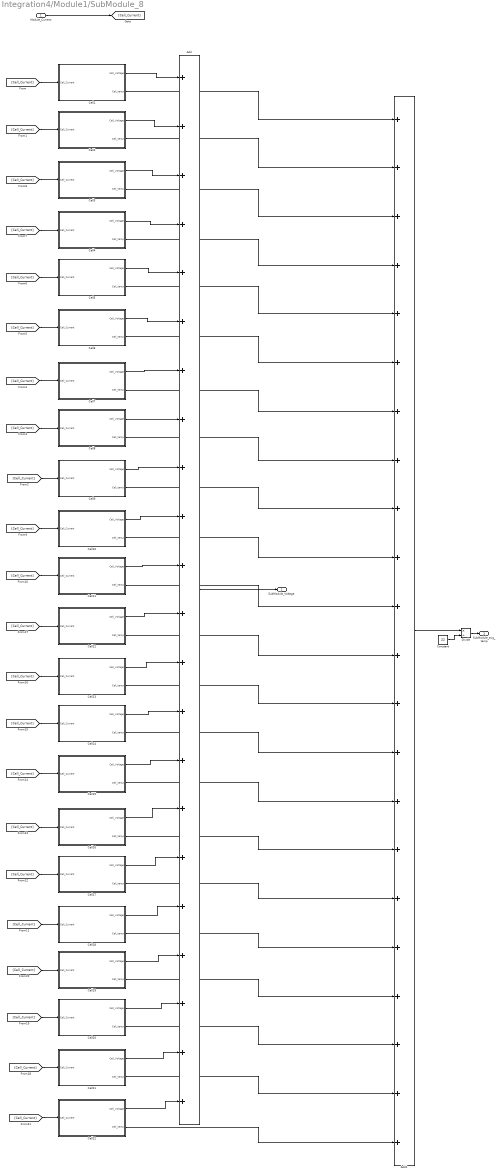
== system Integration4/Module1/SubModule_8 ==
  Module_Current : Inport
  Add : Sum  Inputs=++++++++++++++++++++++
  Add1 : Sum  Inputs=++++++++++++++++++++++
  Cell1 : Subsystem
  Cell10 : Subsystem
  Cell11 : Subsystem
  Cell12 : Subsystem
  Cell13 : Subsystem
  Cell14 : Subsystem
  Cell15 : Subsystem
  Cell16 : Subsystem
  Cell17 : Subsystem
  Cell18 : Subsystem
  Cell19 : Subsystem
  Cell2 : Subsystem
  Cell20 : Subsystem
  Cell21 : Subsystem
  Cell22 : Subsystem
  Cell3 : Subsystem
  Cell4 : Subsystem
  Cell5 : Subsystem
  Cell6 : Subsystem
  Cell7 : Subsystem
  Cell8 : Subsystem
  Cell9 : Subsystem
  Constant : Constant  Value=22
  Divide : Product  Inputs=*/
  SubModule_Voltage : Outport
  SubModule_avg_temp : Outport  Port=2
  wires:
  Cell9/2(Cell_temp) -> Add1/9
  [Cell_Current] -> Cell8/1(Cell_Current)
  Cell13/1(Cell_Voltage) -> Add/13
  Cell4/1(Cell_Voltage) -> Add/4
  Module_Current/1 -> [Cell_Current]
  Cell15/1(Cell_Voltage) -> Add/15
  [Cell_Current] -> Cell7/1(Cell_Current)
  [Cell_Current] -> Cell10/1(Cell_Current)
  Cell21/2(Cell_temp) -> Add1/21
  Cell5/1(Cell_Voltage) -> Add/5
  [Cell_Current] -> Cell1/1(Cell_Current)
  Cell2/1(Cell_Voltage) -> Add/2
  Cell19/1(Cell_Voltage) -> Add/19
  [Cell_Current] -> Cell5/1(Cell_Current)
  [Cell_Current] -> Cell11/1(Cell_Current)
  Cell6/1(Cell_Voltage) -> Add/6
  Cell11/1(Cell_Voltage) -> Add/11
  [Cell_Current] -> Cell18/1(Cell_Current)
  Cell7/2(Cell_temp) -> Add1/7
  [Cell_Current] -> Cell21/1(Cell_Current)
  [Cell_Current] -> Cell12/1(Cell_Current)
  [Cell_Current] -> Cell4/1(Cell_Current)
  Cell18/1(Cell_Voltage) -> Add/18
  Cell20/1(Cell_Voltage) -> Add/20
  Cell11/2(Cell_temp) -> Add1/11
  [Cell_Current] -> Cell2/1(Cell_Current)
  Cell16/2(Cell_temp) -> Add1/16
  [Cell_Current] -> Cell15/1(Cell_Current)
  [Cell_Current] -> Cell6/1(Cell_Current)
  [Cell_Current] -> Cell13/1(Cell_Current)
  Cell2/2(Cell_temp) -> Add1/2
  Cell22/2(Cell_temp) -> Add1/22
  Cell9/1(Cell_Voltage) -> Add/9
  Cell7/1(Cell_Voltage) -> Add/7
  [Cell_Current] -> Cell9/1(Cell_Current)
  Cell14/2(Cell_temp) -> Add1/14
  Cell17/1(Cell_Voltage) -> Add/17
  Cell10/2(Cell_temp) -> Add1/10
  [Cell_Current] -> Cell16/1(Cell_Current)
  Cell8/1(Cell_Voltage) -> Add/8
  Cell21/1(Cell_Voltage) -> Add/21
  Cell12/2(Cell_temp) -> Add1/12
  Cell22/1(Cell_Voltage) -> Add/22
  [Cell_Current] -> Cell20/1(Cell_Current)
  [Cell_Current] -> Cell17/1(Cell_Current)
  Cell10/1(Cell_Voltage) -> Add/10
  Cell18/2(Cell_temp) -> Add1/18
  Cell14/1(Cell_Voltage) -> Add/14
  Cell16/1(Cell_Voltage) -> Add/16
  [Cell_Current] -> Cell3/1(Cell_Current)
  Cell12/1(Cell_Voltage) -> Add/12
  Cell20/2(Cell_temp) -> Add1/20
  Cell1/1(Cell_Voltage) -> Add/1
  [Cell_Current] -> Cell19/1(Cell_Current)
  Cell3/1(Cell_Voltage) -> Add/3
  [Cell_Current] -> Cell22/1(Cell_Current)
  [Cell_Current] -> Cell14/1(Cell_Current)
  Cell19/2(Cell_temp) -> Add1/19
  Cell6/2(Cell_temp) -> Add1/6
  Cell17/2(Cell_temp) -> Add1/17
  Cell15/2(Cell_temp) -> Add1/15
  Cell8/2(Cell_temp) -> Add1/8
  Cell3/2(Cell_temp) -> Add1/3
  Cell13/2(Cell_temp) -> Add1/13
  Add/1 -> SubModule_Voltage/1
  Cell4/2(Cell_temp) -> Add1/4
  Cell5/2(Cell_temp) -> Add1/5
  Cell1/2(Cell_temp) -> Add1/1
  Add1/1 -> Divide/1
  Constant/1 -> Divide/2
  Divide/1 -> SubModule_avg_temp/1
